simulink model "planar_robot_ct_pd_simulation"  (R2014a)
settings: Solver=ode45  StartTime=0.0  StopTime=10  FixedStep=0.0005  MaxStep=0.0005  RelTol=1e-3
values from neighbouring files (symbols this model uses):
  a1 = u_gen(15)    [classical_joint_planar_robot_simulink.m]    (also in ct_gravit_inertia_planar_robot_simulink.m = u_gen(13); ct_gravit_planar_robot_simulink.m = u_gen(13); ct_pid_planar_robot_simulink.m; ct_planar_robot_simulink.m = u_gen(13))
  a2 = u_gen(16)    [classical_joint_planar_robot_simulink.m]    (also in ct_gravit_inertia_planar_robot_simulink.m = u_gen(14); ct_gravit_planar_robot_simulink.m = u_gen(14); ct_pid_planar_robot_simulink.m; ct_planar_robot_simulink.m = u_gen(14))
  b1 = u_gen(17)    [classical_joint_planar_robot_simulink.m]    (also in ct_gravit_inertia_planar_robot_simulink.m = u_gen(15); ct_gravit_planar_robot_simulink.m = u_gen(15); ct_pid_planar_robot_simulink.m; ct_planar_robot_simulink.m = u_gen(15))
  b2 = u_gen(18)    [classical_joint_planar_robot_simulink.m]    (also in ct_gravit_inertia_planar_robot_simulink.m = u_gen(16); ct_gravit_planar_robot_simulink.m = u_gen(16); ct_pid_planar_robot_simulink.m; ct_planar_robot_simulink.m = u_gen(16))
  g = u_gen(19)    [classical_joint_planar_robot_simulink.m]    (also in ct_gravit_inertia_planar_robot_simulink.m = u_gen(17); ct_gravit_planar_robot_simulink.m = u_gen(17); ct_pid_planar_robot_simulink.m; ct_planar_robot_simulink.m = u_gen(17))
  m1 = u_gen(11)    [ac_controller_simulink.m]    (also in classical_joint_planar_robot_simulink.m = u_gen(13); ct_gravit_inertia_planar_robot_simulink.m; ct_gravit_planar_robot_simulink.m; ct_pid_planar_robot_simulink.m = u_gen(13))
  m2 = u_gen(12)    [ac_controller_simulink.m]    (also in classical_joint_planar_robot_simulink.m = u_gen(14); ct_gravit_inertia_planar_robot_simulink.m; ct_gravit_planar_robot_simulink.m; ct_pid_planar_robot_simulink.m = u_gen(14))
settings Model: ExtModeTrigDuration=5000  Creator=Patrick  LastModifiedBy=Patrick
settings SolverCC: PositivePriorityOrder=on
settings RTWCC: SystemTargetFile=quarc_win64.tlc  TemplateMakefile=quarc_default_tmf  Description=QUARC Win64 Target  ProcessScript=quarc_win64_make_rtw_hook
settings STFCustomTargetCC: CombineOutputUpdateFcns=on  GRTInterface=off
settings GRTTargetCC: ParMdlRefBuildCompliant=off  CompOptLevelCompliant=off  MatFileLogging=off  CPPClassGenCompliant=off  ExtMode=on  ExtModeMexFile=quarc_comm

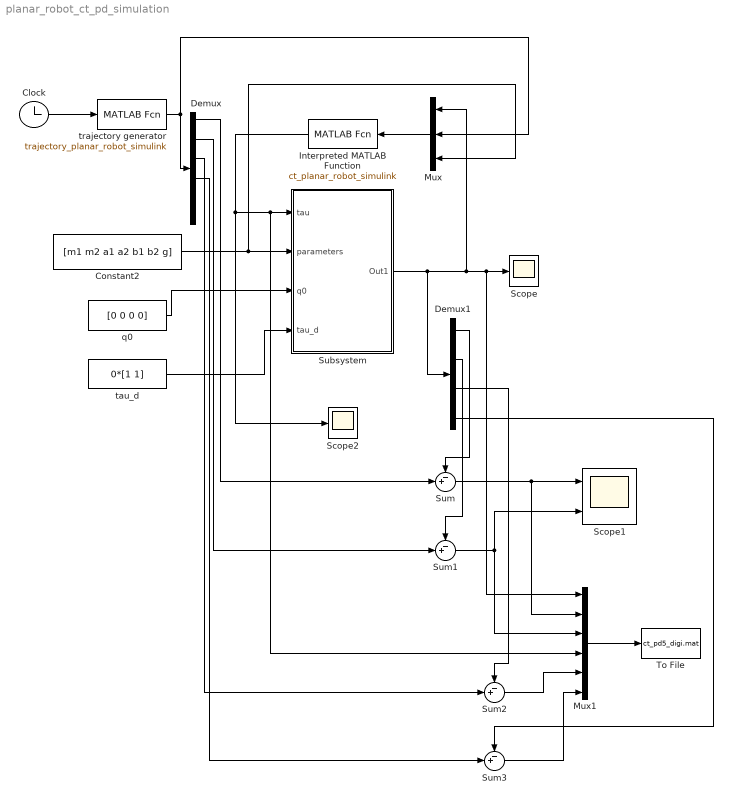
== system planar_robot_ct_pd_simulation ==
  Clock : Clock
  Constant2 : Constant  Value=[m1 m2 a1 a2 b1 b2 g]
  Demux : Demux  Outputs=6
  Demux1 : Demux
  Interpreted MATLAB Function : MATLABFcn  MATLABFcn=ct_planar_robot_simulink  SampleTime=100e-3
  Mux : Mux  Inputs=3
  Mux1 : Mux  Inputs=6
  Scope : Scope
      settings: YMin=-2.75  YMax=2.75
  Scope1 : Scope  NumInputPorts=2
      settings: TimeRange=10  YMin=-0.03~-0.045  YMax=0.03~0.04
  Scope2 : Scope
      settings: YMin=5  YMax=80  SaveName=ScopeData2
  Subsystem : Subsystem
  Sum{,1..3} (4 alike) : Sum  Inputs=-+|
  To File : ToFile  Filename=ct_pd5_digi.mat  MatrixName=ct_pd
  q0 : Constant  Value=[0 0 0 0]
  tau_d : Constant  Value=0*[1 1]
  trajectory generator : MATLABFcn  MATLABFcn=trajectory_planar_robot_simulink
  wires:
  Constant2/1 -> Subsystem/2(parameters), Mux/3
  q0/1 -> Subsystem/3(q0)
  Subsystem/1(Out1) -> Demux1/1, Mux/1, Mux1/1, Scope/1
  Mux/1 -> Interpreted MATLAB Function/1
  Clock/1 -> trajectory generator/1
  trajectory generator/1 -> Demux/1, Mux/2
  Demux/1 -> Sum/2
  Demux1/1 -> Sum/1
  Sum/1 -> Mux1/2, Scope1/1
  Sum1/1 -> Scope1/2, Mux1/3
  Demux1/2 -> Sum1/1
  Demux/2 -> Sum1/2
  Interpreted MATLAB Function/1 -> Scope2/1, Mux1/4, Subsystem/1(tau)
  tau_d/1 -> Subsystem/4(tau_d)
  Mux1/1 -> To File/1
  Sum2/1 -> Mux1/5
  Demux1/3 -> Sum2/1
  Demux1/4 -> Sum3/1
  Sum3/1 -> Mux1/6
  Demux/3 -> Sum2/2
  Demux/4 -> Sum3/2

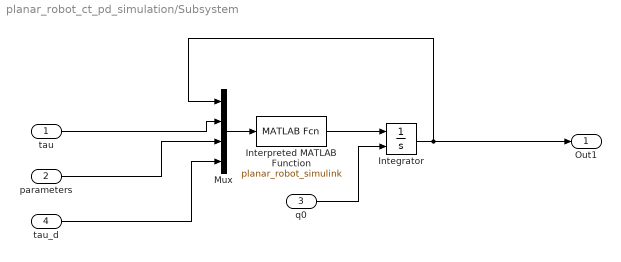
== system planar_robot_ct_pd_simulation/Subsystem ==
  tau : Inport
  parameters : Inport  Port=2
  q0 : Inport  Port=3
  tau_d : Inport  Port=4
  Integrator : Integrator  InitialConditionSource=external
  Interpreted MATLAB Function : MATLABFcn  MATLABFcn=planar_robot_simulink  OutputDimensions=4
  Mux : Mux
  Out1 : Outport
  wires:
  Interpreted MATLAB Function/1 -> Integrator/1
  tau/1 -> Mux/2
  q0/1 -> Integrator/2
  Mux/1 -> Interpreted MATLAB Function/1
  parameters/1 -> Mux/3
  Integrator/1 -> Out1/1, Mux/1
  tau_d/1 -> Mux/4
